simulink model "LFSR"  (R2020a)
settings: Solver=VariableStepAuto  StartTime=0.0  StopTime=10.0  RelTol=1e-3
libraries: simulink_extras x5
settings Model: Creator=kishan  LastModifiedBy=kishan

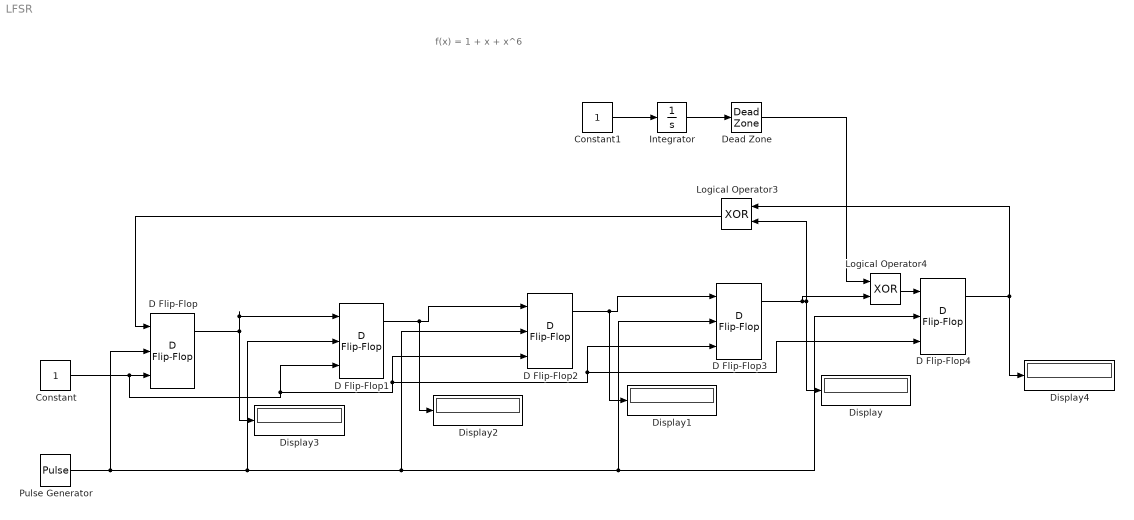
== system LFSR ==
  note: f(x) = 1 + x + x^6
  Constant : Constant
  Constant1 : Constant
  D Flip-Flop{,1..4} (5 alike) : simulink_extras/Flip Flops/D Flip-Flop
  Dead Zone : DeadZone  LowerValue=0.01  UpperValue=10  SaturateOnIntegerOverflow=on
  Display{,1..4} (5 alike) : Display
  Integrator : Integrator
  Logical Operator3 : Logic  Operator=XOR  AllPortsSameDT=off  OutDataTypeStr=boolean
  Logical Operator4 : Logic  Operator=XOR  AllPortsSameDT=off  OutDataTypeStr=boolean
  Pulse Generator : DiscretePulseGenerator  PulseType=Time based  Period=0.01  PulseWidth=5
  wires:
  D Flip-Flop/1 -> D Flip-Flop1/1, Display3/1
  D Flip-Flop1/1 -> D Flip-Flop2/1, Display2/1
  D Flip-Flop2/1 -> D Flip-Flop3/1, Display1/1
  D Flip-Flop3/1 -> Logical Operator4/2, Logical Operator3/2, Display/1
  Logical Operator3/1 -> D Flip-Flop/1
  Pulse Generator/1 -> D Flip-Flop4/2, D Flip-Flop3/2, D Flip-Flop2/2, D Flip-Flop1/2, D Flip-Flop/2
  Constant/1 -> D Flip-Flop4/3, D Flip-Flop3/3, D Flip-Flop2/3, D Flip-Flop1/3, D Flip-Flop/3
  D Flip-Flop4/1 -> Logical Operator3/1, Display4/1
  Logical Operator4/1 -> D Flip-Flop4/1
  Dead Zone/1 -> Logical Operator4/1
  Integrator/1 -> Dead Zone/1
  Constant1/1 -> Integrator/1
